simulink model "n4FFTmodule"  (R2019b)
settings: Solver=VariableStepAuto  StartTime=0.0  StopTime=1  RelTol=1e-3
settings Model: Creator=gjp88  LastModifiedBy=gjp88

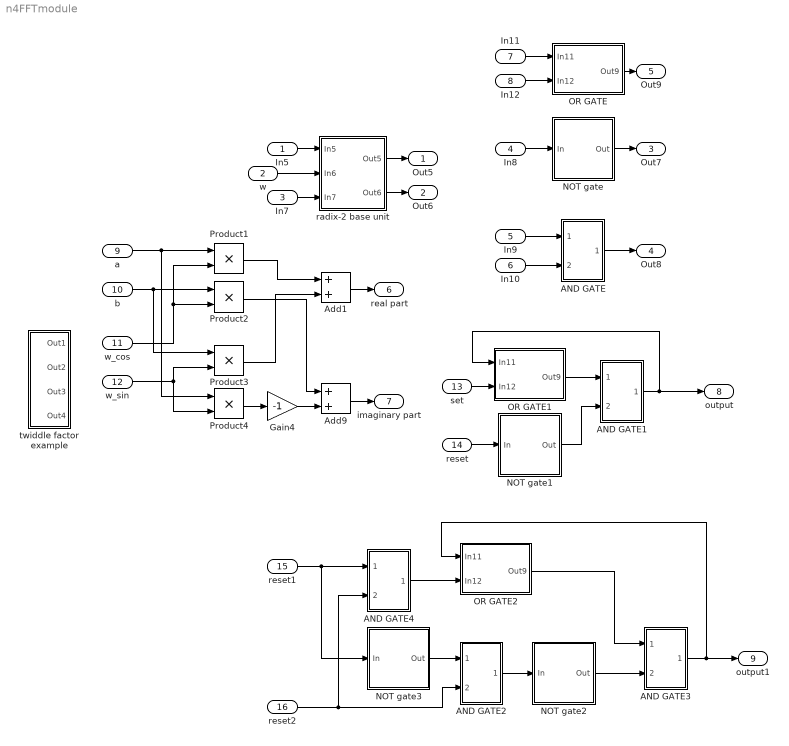
== system n4FFTmodule ==
  In5 : Inport
  w : Inport  Port=2
  In7 : Inport  Port=3
  In8 : Inport  Port=4
  In9 : Inport  Port=5
  In10 : Inport  Port=6
  In11 : Inport  Port=7
  In12 : Inport  Port=8
  a : Inport  Port=9
  b : Inport  Port=10
  w_cos : Inport  Port=11
  w_sin : Inport  Port=12
  set : Inport  Port=13
  reset : Inport  Port=14
  reset1 : Inport  Port=15
  reset2 : Inport  Port=16
  AND GATE : Subsystem
  AND GATE1 : Subsystem
  AND GATE2 : Subsystem
  AND GATE3 : Subsystem
  AND GATE4 : Subsystem
  Add1 : Sum
  Add9 : Sum
  Gain4 : Gain  Gain=-1
  NOT gate : Subsystem
  NOT gate1 : Subsystem
  NOT gate2 : Subsystem
  NOT gate3 : Subsystem
  OR GATE : Subsystem
  OR GATE1 : Subsystem
  OR GATE2 : Subsystem
  Product{1..4} (4 alike) : Product
  radix-2 base unit : Subsystem
  twiddle factor example : Subsystem
  Out5 : Outport
  Out6 : Outport  Port=2
  Out7 : Outport  Port=3
  Out8 : Outport  Port=4
  Out9 : Outport  Port=5
  real part : Outport  Port=6
  imaginary part : Outport  Port=7
  output : Outport  Port=8
  output1 : Outport  Port=9
  wires:
  In8/1 -> NOT gate/1(In)
  NOT gate/1(Out) -> Out7/1
  In9/1 -> AND GATE/1(In9)
  In10/1 -> AND GATE/2(In10)
  AND GATE/1(Out8) -> Out8/1
  In11/1 -> OR GATE/1(In11)
  In12/1 -> OR GATE/2(In12)
  OR GATE/1(Out9) -> Out9/1
  In5/1 -> radix-2 base unit/1(In5)
  w/1 -> radix-2 base unit/2(In6)
  In7/1 -> radix-2 base unit/3(In7)
  radix-2 base unit/1(Out5) -> Out5/1
  radix-2 base unit/2(Out6) -> Out6/1
  a/1 -> Product4/1, Product1/1
  w_cos/1 -> Product2/2, Product1/2
  b/1 -> Product3/1, Product2/1
  w_sin/1 -> Product3/2, Product4/2
  Gain4/1 -> Add9/2
  Product4/1 -> Gain4/1
  Product2/1 -> Add9/1
  Product1/1 -> Add1/1
  Product3/1 -> Add1/2
  Add1/1 -> real part/1
  Add9/1 -> imaginary part/1
  AND GATE1/1(Out8) -> output/1, OR GATE1/1(In11)
  NOT gate1/1(Out) -> AND GATE1/2(In10)
  OR GATE1/1(Out9) -> AND GATE1/1(In9)
  set/1 -> OR GATE1/2(In12)
  reset/1 -> NOT gate1/1(In)
  NOT gate3/1(Out) -> AND GATE2/1(In9)
  reset1/1 -> NOT gate3/1(In), AND GATE4/1(In9)
  reset2/1 -> AND GATE4/2(In10), AND GATE2/2(In10)
  AND GATE2/1(Out8) -> NOT gate2/1(In)
  NOT gate2/1(Out) -> AND GATE3/2(In10)
  AND GATE4/1(Out8) -> OR GATE2/2(In12)
  AND GATE3/1(Out8) -> OR GATE2/1(In11), output1/1
  OR GATE2/1(Out9) -> AND GATE3/1(In9)

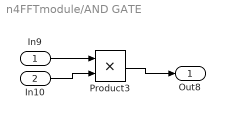
== system n4FFTmodule/AND GATE ==
  In9 : Inport
  In10 : Inport  Port=2
  Product3 : Product
  Out8 : Outport
  wires:
  Product3/1 -> Out8/1
  In9/1 -> Product3/1
  In10/1 -> Product3/2

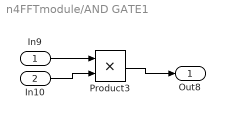
== system n4FFTmodule/AND GATE1 ==
  In9 : Inport
  In10 : Inport  Port=2
  Product3 : Product
  Out8 : Outport
  wires:
  Product3/1 -> Out8/1
  In9/1 -> Product3/1
  In10/1 -> Product3/2

== system n4FFTmodule/AND GATE2 ==
  In9 : Inport
  In10 : Inport  Port=2
  Product3 : Product
  Out8 : Outport
  wires:
  Product3/1 -> Out8/1
  In9/1 -> Product3/1
  In10/1 -> Product3/2

== system n4FFTmodule/AND GATE3 ==
  In9 : Inport
  In10 : Inport  Port=2
  Product3 : Product
  Out8 : Outport
  wires:
  Product3/1 -> Out8/1
  In9/1 -> Product3/1
  In10/1 -> Product3/2

== system n4FFTmodule/AND GATE4 ==
  In9 : Inport
  In10 : Inport  Port=2
  Product3 : Product
  Out8 : Outport
  wires:
  Product3/1 -> Out8/1
  In9/1 -> Product3/1
  In10/1 -> Product3/2

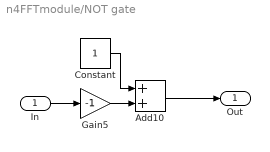
== system n4FFTmodule/NOT gate ==
  In : Inport
  Add10 : Sum
  Constant : Constant
  Gain5 : Gain  Gain=-1
  Out : Outport
  wires:
  Add10/1 -> Out/1
  Gain5/1 -> Add10/2
  In/1 -> Gain5/1
  Constant/1 -> Add10/1

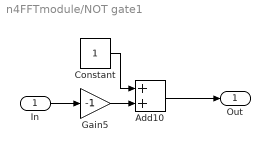
== system n4FFTmodule/NOT gate1 ==
  In : Inport
  Add10 : Sum
  Constant : Constant
  Gain5 : Gain  Gain=-1
  Out : Outport
  wires:
  Add10/1 -> Out/1
  Gain5/1 -> Add10/2
  In/1 -> Gain5/1
  Constant/1 -> Add10/1

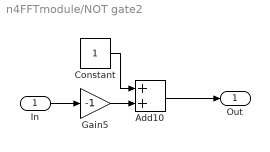
== system n4FFTmodule/NOT gate2 ==
  In : Inport
  Add10 : Sum
  Constant : Constant
  Gain5 : Gain  Gain=-1
  Out : Outport
  wires:
  Add10/1 -> Out/1
  Gain5/1 -> Add10/2
  In/1 -> Gain5/1
  Constant/1 -> Add10/1

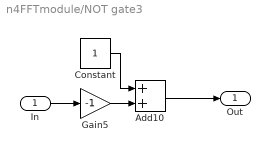
== system n4FFTmodule/NOT gate3 ==
  In : Inport
  Add10 : Sum
  Constant : Constant
  Gain5 : Gain  Gain=-1
  Out : Outport
  wires:
  Add10/1 -> Out/1
  Gain5/1 -> Add10/2
  In/1 -> Gain5/1
  Constant/1 -> Add10/1

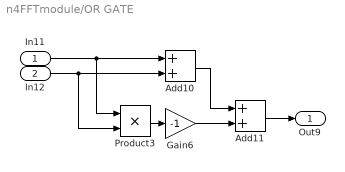
== system n4FFTmodule/OR GATE ==
  In11 : Inport
  In12 : Inport  Port=2
  Add10 : Sum
  Add11 : Sum
  Gain6 : Gain  Gain=-1
  Product3 : Product
  Out9 : Outport
  wires:
  In12/1 -> Product3/2, Add10/2
  Gain6/1 -> Add11/2
  Product3/1 -> Gain6/1
  In11/1 -> Product3/1, Add10/1
  Add11/1 -> Out9/1
  Add10/1 -> Add11/1

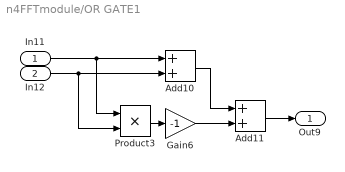
== system n4FFTmodule/OR GATE1 ==
  In11 : Inport
  In12 : Inport  Port=2
  Add10 : Sum
  Add11 : Sum
  Gain6 : Gain  Gain=-1
  Product3 : Product
  Out9 : Outport
  wires:
  In12/1 -> Product3/2, Add10/2
  Gain6/1 -> Add11/2
  Product3/1 -> Gain6/1
  In11/1 -> Product3/1, Add10/1
  Add11/1 -> Out9/1
  Add10/1 -> Add11/1

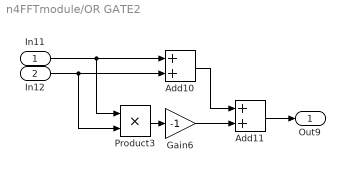
== system n4FFTmodule/OR GATE2 ==
  In11 : Inport
  In12 : Inport  Port=2
  Add10 : Sum
  Add11 : Sum
  Gain6 : Gain  Gain=-1
  Product3 : Product
  Out9 : Outport
  wires:
  In12/1 -> Product3/2, Add10/2
  Gain6/1 -> Add11/2
  Product3/1 -> Gain6/1
  In11/1 -> Product3/1, Add10/1
  Add11/1 -> Out9/1
  Add10/1 -> Add11/1

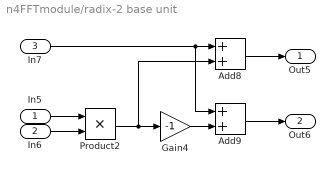
== system n4FFTmodule/radix-2 base unit ==
  In5 : Inport
  In6 : Inport  Port=2
  In7 : Inport  Port=3
  Add8 : Sum
  Add9 : Sum
  Gain4 : Gain  Gain=-1
  Product2 : Product
  Out5 : Outport
  Out6 : Outport  Port=2
  wires:
  In5/1 -> Product2/1
  In7/1 -> Add9/1, Add8/1
  Gain4/1 -> Add9/2
  Add8/1 -> Out5/1
  In6/1 -> Product2/2
  Add9/1 -> Out6/1
  Product2/1 -> Gain4/1, Add8/2

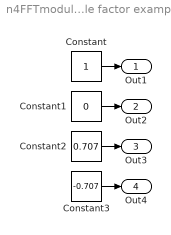
== system n4FFTmodule/twiddle factor example ==
  Constant : Constant
  Constant1 : Constant  Value=0
  Constant2 : Constant  Value=0.707
  Constant3 : Constant  Value=-0.707
  Out1 : Outport
  Out2 : Outport  Port=2
  Out3 : Outport  Port=3
  Out4 : Outport  Port=4
  wires:
  Constant/1 -> Out1/1
  Constant1/1 -> Out2/1
  Constant3/1 -> Out4/1
  Constant2/1 -> Out3/1
